simulink model "PV_RT_PI_FDI_DoS_2017b"  (R2017b)
settings: Solver=ode23tb  StartTime=0.0  StopTime=30  FixedStep=0.1  RelTol=1e-3
values from neighbouring files (symbols this model uses):
  DoS1 = data.DoS1(i)    [CyberAttack_Performance.m]
  DoS2 = data.DoS2(i)    [CyberAttack_Performance.m]
  FDI1 = data.FDI1(i)    [CyberAttack_Performance.m]
  FDI2 = data.FDI2(i)    [CyberAttack_Performance.m]
  Ki1 = 0.4024    [CyberAttack_Performance.m]
  Ki2 = 0.7256    [CyberAttack_Performance.m]
  Kp1 = 0.5663    [CyberAttack_Performance.m]
  Kp2 = 0.5127    [CyberAttack_Performance.m]
  SLP2 = data.SLP2(i)    [CyberAttack_Performance.m]
undefined symbols (not defined in the file or in its folder): a1, B1, b1, c1, d1, Kd, Kps1, Kr1, R1, T12, Tg1, Tps1, Tr1, Tt1
libraries: simulink x2
settings Model: Creator=Fujitsu  LastModifiedBy=bora_
settings SolverCC: ZeroCrossAlgorithm=Adaptive
settings DataIOCC: MaxDataPoints=10  SaveFormat=Array  SaveOutput=off  SignalLogging=off  DSMLogging=off  SaveTime=off
settings OptimizationCC: EfficientMapNaN2IntZero=off
settings HardwareCC: TargetBitPerPointer=64  TargetBitPerSizeT=64  TargetBitPerPtrDiffT=64  TargetLongLongMode=on  TargetIntDivRoundTo=Zero  TargetEndianess=LittleEndian  TargetWordSize=64  TargetHWDeviceType=MATLAB Host  ProdEqTarget=off
settings CodeAppCC: MaxIdLength=128
settings GRTTargetCC: TargetLangStandard=C89/C90 (ANSI)  CombineOutputUpdateFcns=off  GRTInterface=on

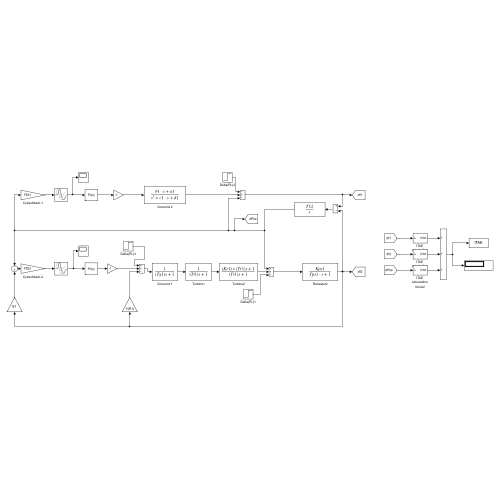
[thumbnail: Simulink's stored preview of the top-level diagram]
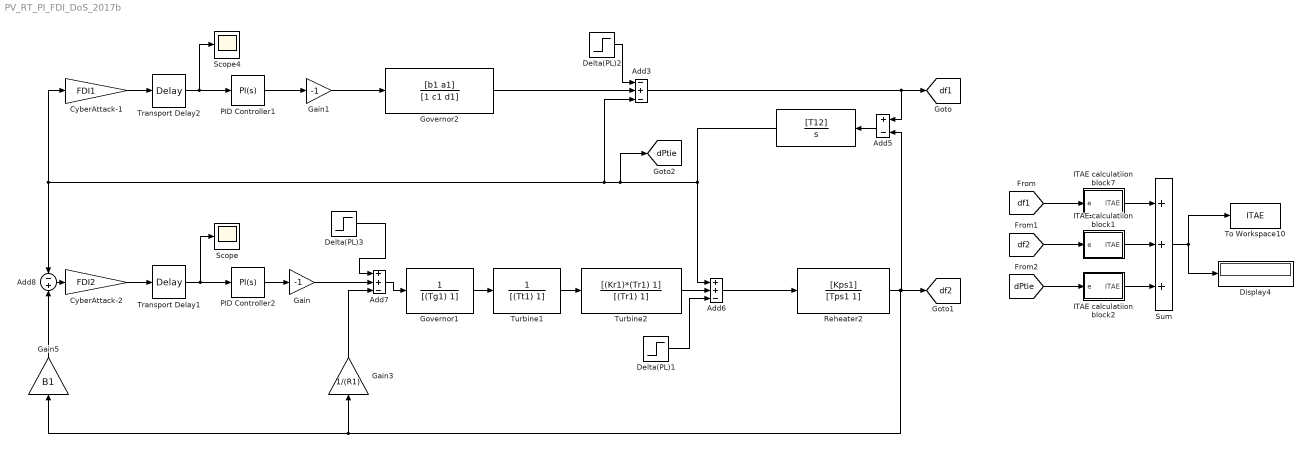
== system PV_RT_PI_FDI_DoS_2017b ==
  " " : TransferFcn  Numerator=[T12]  Denominator=[1 0]
  Add3 : Sum  Inputs=-+-
  Add5 : Sum  Inputs=+-
  Add6 : Sum  Inputs=++-
  Add7 : Sum  Inputs=++-
  Add8 : Sum  Inputs=-+
  CyberAttack-1 : Gain  Gain=FDI1
  CyberAttack-2 : Gain  Gain=FDI2
  Delta(PL)1 : Step  Time=0  After=SLP2  SampleTime=0.1
  Delta(PL)2 : Step  Time=0  After=0  SampleTime=0.1
  Delta(PL)3 : Step  Time=0  After=0  SampleTime=0.1
  Display4 : Display
  Gain : Gain  Gain=-1
  Gain1 : Gain  Gain=-1
  Gain3 : Gain  Gain=1/(R1)
  Gain5 : Gain  Gain=B1
  Governor1 : TransferFcn  Denominator=[(Tg1) 1]
  Governor2 : TransferFcn  Numerator=[b1 a1]  Denominator=[1 c1 d1]
  ITAE calculatiion block1 : Subsystem
  ITAE calculatiion block2 : Subsystem
  ITAE calculatiion block7 : Subsystem
  PID Controller1 : simulink/Continuous/PID Controller  Controller=PI  Form=Parallel  TimeDomain=Continuous-time  SampleTime=-1  IntegratorMethod=Forward Euler  ControllerParametersSource=internal  P=Kp1  I=Ki1  D=Kd  N=1000000  UseFilter=on  TunerSelectOption=Transfer Function Based (PID Tuner App)  InitialConditionSource=internal  InitialConditionForIntegrator=0  InitialConditionForFilter=0  DifferentiatorICPrevScaledInput=0  ExternalReset=none  TrackingMode=off  Kt=1  LimitOutput=off  UpperSaturationLimit=inf  LowerSaturationLimit=-inf  LinearizeAsGain=on  AntiWindupMode=none  Kb=1  POutMin=[]  POutMax=[]  IOutMin=[]  IOutMax=[]  DOutMin=[]  DOutMax=[]  NOutMin=[]  NOutMax=[]  SumOutMin=[]  SumOutMax=[]  SaturationOutMin=[]  SaturationOutMax=[]  PParamMin=[]  PParamMax=[]  IParamMin=[]  IParamMax=[]  DParamMin=[]  DParamMax=[]  NParamMin=[]  NParamMax=[]  KbParamMin=[]  KbParamMax=[]  KtParamMin=[]  KtParamMax=[]  KbOutMin=[]  KbOutMax=[]  KtOutMin=[]  KtOutMax=[]  IntegratorOutMin=[]  IntegratorOutMax=[]  FilterOutMin=[]  FilterOutMax=[]  SumI1OutMin=[]  SumI1OutMax=[]  SumI2OutMin=[]  SumI2OutMax=[]  SumI3OutMin=[]  SumI3OutMax=[]  SumDOutMin=[]  SumDOutMax=[]  DifferentiatorOutMin=[]  DifferentiatorOutMax=[]  FilterDiffOutCoefMin=[]  FilterDiffOutCoefMax=[]  ReciprocalOutMin=[]  ReciprocalOutMax=[]  SumDenOutMin=[]  SumDenOutMax=[]  SumNumOutMin=[]  SumNumOutMax=[]  DivideOutMin=[]  DivideOutMax=[]  IntegratorContinuousStateAttributes=''  IntegratorStateMustResolveToSignalObject=off  IntegratorRTWStateStorageClass=Auto  FilterContinuousStateAttributes=''  FilterStateMustResolveToSignalObject=off  FilterRTWStateStorageClass=Auto  InitialConditionSetting=State (most efficient)
  PID Controller2 : simulink/Continuous/PID Controller  Controller=PI  Form=Parallel  TimeDomain=Continuous-time  SampleTime=-1  IntegratorMethod=Forward Euler  ControllerParametersSource=internal  P=Kp2  I=Ki2  D=Kd  N=1000000  UseFilter=on  TunerSelectOption=Transfer Function Based (PID Tuner App)  InitialConditionSource=internal  InitialConditionForIntegrator=0  InitialConditionForFilter=0  DifferentiatorICPrevScaledInput=0  ExternalReset=none  TrackingMode=off  Kt=1  LimitOutput=off  UpperSaturationLimit=inf  LowerSaturationLimit=-inf  LinearizeAsGain=on  AntiWindupMode=none  Kb=1  POutMin=[]  POutMax=[]  IOutMin=[]  IOutMax=[]  DOutMin=[]  DOutMax=[]  NOutMin=[]  NOutMax=[]  SumOutMin=[]  SumOutMax=[]  SaturationOutMin=[]  SaturationOutMax=[]  PParamMin=[]  PParamMax=[]  IParamMin=[]  IParamMax=[]  DParamMin=[]  DParamMax=[]  NParamMin=[]  NParamMax=[]  KbParamMin=[]  KbParamMax=[]  KtParamMin=[]  KtParamMax=[]  KbOutMin=[]  KbOutMax=[]  KtOutMin=[]  KtOutMax=[]  IntegratorOutMin=[]  IntegratorOutMax=[]  FilterOutMin=[]  FilterOutMax=[]  SumI1OutMin=[]  SumI1OutMax=[]  SumI2OutMin=[]  SumI2OutMax=[]  SumI3OutMin=[]  SumI3OutMax=[]  SumDOutMin=[]  SumDOutMax=[]  DifferentiatorOutMin=[]  DifferentiatorOutMax=[]  FilterDiffOutCoefMin=[]  FilterDiffOutCoefMax=[]  ReciprocalOutMin=[]  ReciprocalOutMax=[]  SumDenOutMin=[]  SumDenOutMax=[]  SumNumOutMin=[]  SumNumOutMax=[]  DivideOutMin=[]  DivideOutMax=[]  IntegratorContinuousStateAttributes=''  IntegratorStateMustResolveToSignalObject=off  IntegratorRTWStateStorageClass=Auto  FilterContinuousStateAttributes=''  FilterStateMustResolveToSignalObject=off  FilterRTWStateStorageClass=Auto  InitialConditionSetting=State (most efficient)
  Reheater2 : TransferFcn  Numerator=[Kps1]  Denominator=[Tps1 1]
  Scope : Scope
  Scope4 : Scope
  Sum : Sum  Inputs=+++
  To Workspace10 : ToWorkspace  VariableName=ITAE  SampleTime=0.1
      settings: Save2DSignal=2-D array (concatenate along first dimension)
  Transport Delay1 : TransportDelay  DelayTime=DoS2
  Transport Delay2 : TransportDelay  DelayTime=DoS1
  Turbine1 : TransferFcn  Denominator=[(Tt1) 1]
  Turbine2 : TransferFcn  Numerator=[(Kr1)*(Tr1) 1]  Denominator=[(Tr1) 1]
  tag scope: dPtie=global, df1=global, df2=global
  wires:
  " "/1 -> Add6/1, Add3/3, CyberAttack-1/1, Add8/1, [dPtie]
  Gain5/1 -> Add8/2
  Reheater2/1 -> [df2], Add5/2, Gain5/1, Gain3/1
  Gain3/1 -> Add7/3
  Delta(PL)1/1 -> Add6/3
  Turbine1/1 -> Turbine2/1
  Governor1/1 -> Turbine1/1
  Add5/1 -> " "/1
  Add7/1 -> Governor1/1
  Turbine2/1 -> Add6/2
  PID Controller1/1 -> Gain1/1
  Governor2/1 -> Add3/2
  Delta(PL)2/1 -> Add3/1
  PID Controller2/1 -> Gain/1
  Delta(PL)3/1 -> Add7/1
  Gain1/1 -> Governor2/1
  Gain/1 -> Add7/2
  Add3/1 -> [df1], Add5/1
  Add6/1 -> Reheater2/1
  [df1] -> ITAE calculatiion block7/1(e)
  ITAE calculatiion block1/1(ITAE) -> Sum/2
  [dPtie] -> ITAE calculatiion block2/1(e)
  ITAE calculatiion block7/1(ITAE) -> Sum/1
  ITAE calculatiion block2/1(ITAE) -> Sum/3
  [df2] -> ITAE calculatiion block1/1(e)
  Sum/1 -> To Workspace10/1, Display4/1
  CyberAttack-1/1 -> Transport Delay2/1
  Add8/1 -> CyberAttack-2/1
  CyberAttack-2/1 -> Transport Delay1/1
  Transport Delay1/1 -> PID Controller2/1, Scope/1
  Transport Delay2/1 -> PID Controller1/1, Scope4/1

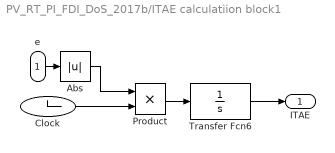
== system PV_RT_PI_FDI_DoS_2017b/ITAE calculatiion block1 ==
  e : Inport
  Abs : Abs  ZeroCross=off
  Clock : Clock
  Product : Product  RndMeth=Zero
  Transfer Fcn6 : TransferFcn  Denominator=[1 0]
  ITAE : Outport  VectorParamsAs1DForOutWhenUnconnected=off
  wires:
  e/1 -> Abs/1
  Clock/1 -> Product/2
  Abs/1 -> Product/1
  Transfer Fcn6/1 -> ITAE/1
  Product/1 -> Transfer Fcn6/1

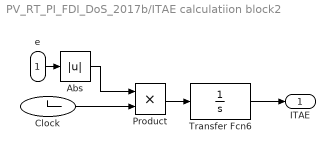
== system PV_RT_PI_FDI_DoS_2017b/ITAE calculatiion block2 ==
  e : Inport
  Abs : Abs  ZeroCross=off
  Clock : Clock
  Product : Product  RndMeth=Zero
  Transfer Fcn6 : TransferFcn  Denominator=[1 0]
  ITAE : Outport  VectorParamsAs1DForOutWhenUnconnected=off
  wires:
  Product/1 -> Transfer Fcn6/1
  Transfer Fcn6/1 -> ITAE/1
  Abs/1 -> Product/1
  Clock/1 -> Product/2
  e/1 -> Abs/1

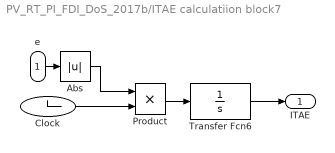
== system PV_RT_PI_FDI_DoS_2017b/ITAE calculatiion block7 ==
  e : Inport
  Abs : Abs  ZeroCross=off
  Clock : Clock
  Product : Product  RndMeth=Zero
  Transfer Fcn6 : TransferFcn  Denominator=[1 0]
  ITAE : Outport  VectorParamsAs1DForOutWhenUnconnected=off
  wires:
  Product/1 -> Transfer Fcn6/1
  Transfer Fcn6/1 -> ITAE/1
  Abs/1 -> Product/1
  Clock/1 -> Product/2
  e/1 -> Abs/1
